simulink model "PassangerVehicle"  (R2022a)
settings: Solver=ode23tb  StartTime=0.0  StopTime=15  RelTol=1e-3
values from neighbouring files (symbols this model uses):
  AccPwrbp = [0 3.0779560993538198]    [Init_Parameters.m]
  AccSpdbp = [256.49641719585139 641.24104298962845]    [Init_Parameters.m]
  InitialLatPosition = 0    [Init_Parameters.m]
  numWheels = 4    [Init_Parameters.m]    (also in VehicleParameters.m)
  TrackWidth = VEH.TrackWidth    [Init_Parameters.m]
  Trans = data.Trans    [Init_Parameters.m]    (also in ModelWorkspace.mat = )
  VEH = data.VEH    [Init_Parameters.m]    (also in ModelWorkspace.mat = ; VehicleParameters.m)
  wheelB = VEH.FrontAxlePositionfromCG+VEH.RearAxlePositionfromCG    [Init_Parameters.m]    (also in VehicleParameters.m)
libraries: autolibutils x6, sharedtransform x5, autolibsharedcoupling x3, vehdynlibsuspension x2, shared6dof x2, autolibsharedtransfixedgear x1, vehdynlibsteering x1, autolibshareddiff x1, autolibsharedmappedengines x1, vehdynlibeom x1, vehdynlibtire x1, vehdynlibtirecommon x1
(part 1 of 4)
settings Model: Creator=monic  LastModifiedBy=monic
settings DebuggingCC: UnconnectedInputMsg=warning  UnconnectedOutputMsg=warning  UnconnectedLineMsg=warning
settings RTWCC: DLArmComputeVersion=19.05

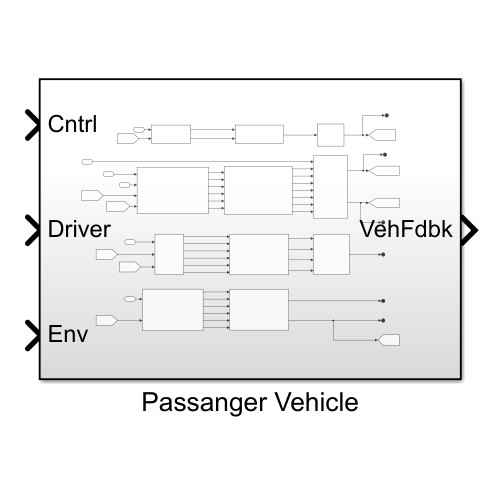
[thumbnail: Simulink's stored preview of the top-level diagram]
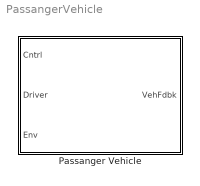
== system PassangerVehicle ==
  Passanger Vehicle : Subsystem

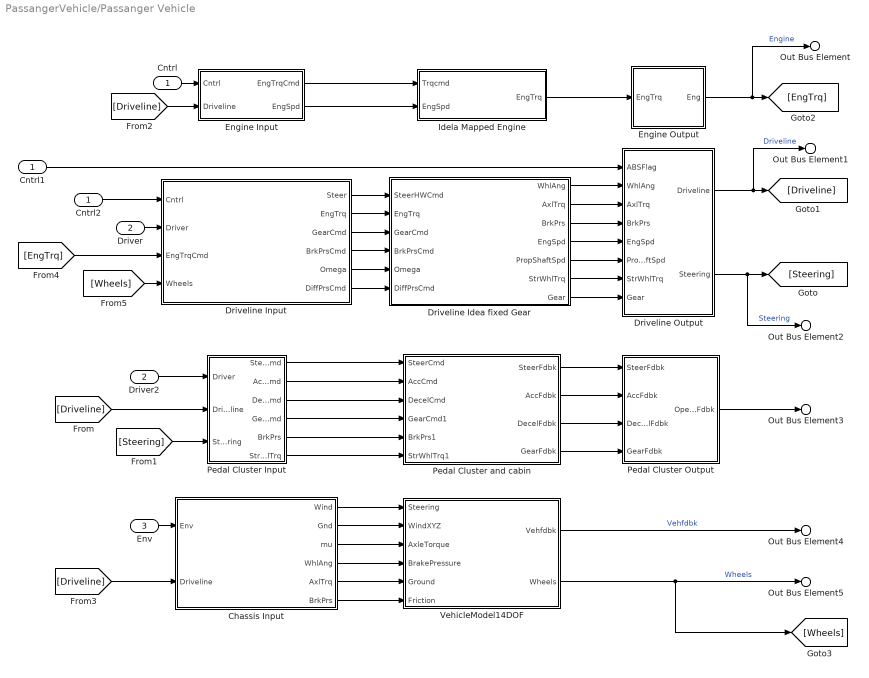
== system PassangerVehicle/Passanger Vehicle ==
  Cntrl : Inport
  Driver : Inport  Port=2
  Env : Inport  Port=3
  Chassis Input : Subsystem
  Cntrl1 : InportShadow
  Cntrl2 : InportShadow
  Driveline Idea fixed Gear : Subsystem
  Driveline Input : Subsystem
  Driveline Output : Subsystem
  Driver2 : InportShadow  Port=2
  Engine Input : Subsystem
  Engine Output : Subsystem
  Idela Mapped Engine : Subsystem
  Pedal Cluster Input : Subsystem
  Pedal Cluster Output : Subsystem
  Pedal Cluster and cabin : Subsystem
  VehicleModel14DOF : Subsystem
  Out Bus Element4 : Outport  PortName=VehFdbk  Element=Body
  Out Bus Element5 : Outport  PortName=VehFdbk  Element=Wheels
  Out Bus Element3 : Outport  PortName=VehFdbk  Element=Driver
  Out Bus Element2 : Outport  PortName=VehFdbk  Element=Steering
  Out Bus Element1 : Outport  PortName=VehFdbk  Element=Driveline
  Out Bus Element : Outport  PortName=VehFdbk  Element=Engine
  wires:
  Driveline Idea fixed Gear/7(Gear) -> Driveline Output/8(Gear)
  [Driveline] -> Chassis Input/2(Driveline)
  Engine Input/1(EngTrqCmd) -> Idela Mapped Engine/1(Trqcmd)
  Pedal Cluster and cabin/2(AccFdbk) -> Pedal Cluster Output/2(AccFdbk)
  Chassis Input/6(BrkPrs) -> VehicleModel14DOF/6(Friction)
  Driveline Input/4(BrkPrsCmd) -> Driveline Idea fixed Gear/4(BrkPrsCmd)
  Pedal Cluster Input/3(DecelCmd) -> Pedal Cluster and cabin/3(DecelCmd)
  VehicleModel14DOF/2(Wheels) -> Out Bus Element5/1, [Wheels]  "Wheels"
  Chassis Input/4(WhlAng) -> VehicleModel14DOF/4(BrakePressure)
  Pedal Cluster Input/2(AccelCmd) -> Pedal Cluster and cabin/2(AccCmd)
  Driver/1 -> Driveline Input/2(Driver)
  Pedal Cluster and cabin/3(DecelFdbk) -> Pedal Cluster Output/3(DecelFdbk)
  Engine Input/2(EngSpd) -> Idela Mapped Engine/2(EngSpd)
  [Driveline] -> Pedal Cluster Input/2(Driveline)
  Driveline Idea fixed Gear/1(WhlAng) -> Driveline Output/2(WhlAng)
  Pedal Cluster and cabin/4(GearFdbk) -> Pedal Cluster Output/4(GearFdbk)
  Driveline Input/3(GearCmd) -> Driveline Idea fixed Gear/3(GearCmd)
  [Steering] -> Pedal Cluster Input/3(Steering)
  Cntrl1/1 -> Driveline Output/1(ABSFlag)
  [EngTrq] -> Driveline Input/3(EngTrqCmd)
  Chassis Input/3(mu) -> VehicleModel14DOF/3(AxleTorque)
  Chassis Input/5(AxlTrq) -> VehicleModel14DOF/5(Ground)
  Driveline Input/6(DiffPrsCmd) -> Driveline Idea fixed Gear/6(DiffPrsCmd)
  Driver2/1 -> Pedal Cluster Input/1(Driver)
  Idela Mapped Engine/1(EngTrq) -> Engine Output/1("EngTrq ")
  Pedal Cluster Input/1(SteerCmd) -> Pedal Cluster and cabin/1(SteerCmd)
  Cntrl/1 -> Engine Input/1(Cntrl)
  Pedal Cluster Input/5(BrkPrs) -> Pedal Cluster and cabin/5(BrkPrs1)
  [Wheels] -> Driveline Input/4(Wheels)
  Driveline Input/1(Steer) -> Driveline Idea fixed Gear/1(SteerHWCmd)
  Driveline Input/2(EngTrq) -> Driveline Idea fixed Gear/2(EngTrq)
  Pedal Cluster and cabin/1(SteerFdbk) -> Pedal Cluster Output/1(SteerFdbk)
  Driveline Input/5(Omega) -> Driveline Idea fixed Gear/5(Omega)
  Env/1 -> Chassis Input/1(Env)
  Driveline Idea fixed Gear/3(BrkPrs) -> Driveline Output/4(BrkPrs)
  Chassis Input/1(Wind) -> VehicleModel14DOF/1(Steering)
  Driveline Idea fixed Gear/4(EngSpd) -> Driveline Output/5(EngSpd)
  Chassis Input/2(Gnd) -> VehicleModel14DOF/2(WindXYZ)
  Driveline Output/2(Steering) -> Out Bus Element2/1, [Steering]  "Steering"
  Engine Output/1(Eng) -> Out Bus Element/1, [EngTrq]  "Engine"
  Driveline Idea fixed Gear/6(StrWhlTrq) -> Driveline Output/7(StrWhlTrq)
  Driveline Idea fixed Gear/5(PropShaftSpd) -> Driveline Output/6(PropShftSpd)
  [Driveline] -> Engine Input/2(Driveline)
  Pedal Cluster Input/4(GearCmd) -> Pedal Cluster and cabin/4(GearCmd1)
  Driveline Idea fixed Gear/2(AxlTrq) -> Driveline Output/3(AxlTrq)
  VehicleModel14DOF/1(Vehfdbk) -> Out Bus Element4/1  "Vehfdbk"
  Pedal Cluster Input/6(StrWhlTrq) -> Pedal Cluster and cabin/6(StrWhlTrq1)
  Cntrl2/1 -> Driveline Input/1(Cntrl)
  Pedal Cluster Output/1(OperatorFdbk) -> Out Bus Element3/1
  Driveline Output/1(Driveline) -> Out Bus Element1/1, [Driveline]  "Driveline"

== system PassangerVehicle/Passanger Vehicle/Chassis Input ==
  Env : Inport
  Driveline : Inport  Port=2
  Bus Selector1 : BusSelector  OutputSignals=Gnd.z.G_FL_z,Gnd.z.G_FR_z,Gnd.z.G_RL_z,Gnd.z.G_RR_z
  Bus Selector2 : BusSelector  OutputSignals=Wind
  Bus Selector3 : BusSelector  OutputSignals=Gnd.mu.mu_FL,Gnd.mu.mu_FR,Gnd.mu.mu_RL,Gnd.mu.mu_RR
  Bus Selector4 : BusSelector  OutputSignals=WhlAng,AxlTrq,BrkPrs
  Vector Concatenate : Concatenate  NumInputs=4
  Vector Concatenate1 : Concatenate  NumInputs=4
  Wind : Outport  VectorParamsAs1DForOutWhenUnconnected=off
  Gnd : Outport  Port=2  VectorParamsAs1DForOutWhenUnconnected=off
  mu : Outport  Port=3  VectorParamsAs1DForOutWhenUnconnected=off
  WhlAng : Outport  Port=4  VectorParamsAs1DForOutWhenUnconnected=off
  AxlTrq : Outport  Port=5  VectorParamsAs1DForOutWhenUnconnected=off
  BrkPrs : Outport  Port=6  VectorParamsAs1DForOutWhenUnconnected=off
  wires:
  Env/1 -> Bus Selector3/1, Bus Selector1/1, Bus Selector2/1
  Bus Selector2/1 -> Wind/1  "<Wind>"
  Bus Selector3/1 -> Vector Concatenate/1  "<mu_FL>"
  Bus Selector3/2 -> Vector Concatenate/2  "<mu_FR>"
  Bus Selector3/3 -> Vector Concatenate/3  "<mu_RL>"
  Bus Selector3/4 -> Vector Concatenate/4  "<mu_RR>"
  Vector Concatenate/1 -> mu/1
  Bus Selector1/1 -> Vector Concatenate1/1  "<G_FL_z>"
  Bus Selector1/2 -> Vector Concatenate1/2  "<G_FR_z>"
  Bus Selector1/3 -> Vector Concatenate1/3  "<G_RL_z>"
  Bus Selector1/4 -> Vector Concatenate1/4  "<G_RR_z>"
  Vector Concatenate1/1 -> Gnd/1
  Driveline/1 -> Bus Selector4/1
  Bus Selector4/2 -> AxlTrq/1  "<AxlTrq>"
  Bus Selector4/1 -> WhlAng/1  "<WhlAng>"
  Bus Selector4/3 -> BrkPrs/1  "<BrkPrs>"

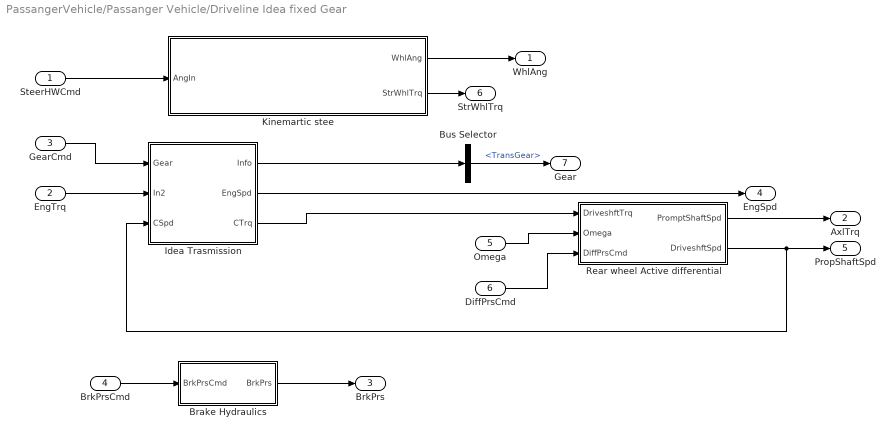
== system PassangerVehicle/Passanger Vehicle/Driveline Idea fixed Gear ==
  SteerHWCmd : Inport
  EngTrq : Inport  Port=2
  GearCmd : Inport  Port=3
  BrkPrsCmd : Inport  Port=4  PortDimensions=4
  Omega : Inport  Port=5
  DiffPrsCmd : Inport  Port=6
  Brake Hydraulics : Subsystem
  Bus Selector : BusSelector  OutputSignals=Trans.TransGear
  Idea Trasmission : Subsystem
  Kinemartic stee : Subsystem
  Rear wheel Active differential : Subsystem
  WhlAng : Outport  Unit=rad  VectorParamsAs1DForOutWhenUnconnected=off
  AxlTrq : Outport  Port=2  VectorParamsAs1DForOutWhenUnconnected=off
  BrkPrs : Outport  Port=3  PortDimensions=4  VectorParamsAs1DForOutWhenUnconnected=off
  EngSpd : Outport  Port=4  VectorParamsAs1DForOutWhenUnconnected=off
  PropShaftSpd : Outport  Port=5  VectorParamsAs1DForOutWhenUnconnected=off
  StrWhlTrq : Outport  Port=6  Unit=N*m  VectorParamsAs1DForOutWhenUnconnected=off
  Gear : Outport  Port=7
  wires:
  Rear wheel Active differential/1(PromptShaftSpd) -> AxlTrq/1
  Omega/1 -> Rear wheel Active differential/2(Omega)
  Rear wheel Active differential/2(DriveshftSpd) -> PropShaftSpd/1, Idea Trasmission/3(CSpd)
  Idea Trasmission/3(CTrq) -> Rear wheel Active differential/1(DriveshftTrq)
  DiffPrsCmd/1 -> Rear wheel Active differential/3(DiffPrsCmd)
  Brake Hydraulics/1(BrkPrs) -> BrkPrs/1
  Idea Trasmission/2(EngSpd) -> EngSpd/1
  BrkPrsCmd/1 -> Brake Hydraulics/1(BrkPrsCmd)
  GearCmd/1 -> Idea Trasmission/1(Gear)
  SteerHWCmd/1 -> Kinemartic stee/1(AngIn)
  Idea Trasmission/1(Info) -> Bus Selector/1
  Kinemartic stee/2(StrWhlTrq) -> StrWhlTrq/1
  Kinemartic stee/1(WhlAng) -> WhlAng/1
  EngTrq/1 -> Idea Trasmission/2(In2)
  Bus Selector/1 -> Gear/1  "<TransGear>"

== system PassangerVehicle/Passanger Vehicle/Driveline Input ==
  Cntrl : Inport
  Driver : Inport  Port=2
  EngTrqCmd : Inport  Port=3
  Wheels : Inport  Port=4
  Bus Selector1 : BusSelector  OutputSignals=SteerCmd
  Bus Selector2 : BusSelector  OutputSignals=TireFrame.Omega
  Bus Selector3 : BusSelector  OutputSignals=Transmission.GearCmd,Brake.BrkPrsCmd,Diff.DiffPrsCmd
  Bus Selector4 : BusSelector  OutputSignals=EngTrq
  Data Type Conversion : DataTypeConversion  SaturateOnIntegerOverflow=off  RndMeth=Floor
  Steer : Outport  VectorParamsAs1DForOutWhenUnconnected=off
  EngTrq : Outport  Port=2  VectorParamsAs1DForOutWhenUnconnected=off
  GearCmd : Outport  Port=3  VectorParamsAs1DForOutWhenUnconnected=off
  BrkPrsCmd : Outport  Port=4  VectorParamsAs1DForOutWhenUnconnected=off
  Omega : Outport  Port=5  VectorParamsAs1DForOutWhenUnconnected=off
  DiffPrsCmd : Outport  Port=6  VectorParamsAs1DForOutWhenUnconnected=off
  wires:
  Cntrl/1 -> Bus Selector3/1
  Bus Selector3/1 -> Data Type Conversion/1  "<GearCmd>"
  Driver/1 -> Bus Selector1/1
  Wheels/1 -> Bus Selector2/1
  Bus Selector2/1 -> Omega/1  "<Omega>"
  Bus Selector3/2 -> BrkPrsCmd/1  "<BrkPrsCmd>"
  EngTrqCmd/1 -> Bus Selector4/1
  Bus Selector1/1 -> Steer/1  "<SteerCmd>"
  Bus Selector4/1 -> EngTrq/1  "<EngTrq>"
  Bus Selector3/3 -> DiffPrsCmd/1  "<DiffPrsCmd>"
  Data Type Conversion/1 -> GearCmd/1

== system PassangerVehicle/Passanger Vehicle/Driveline Output ==
  ABSFlag : Inport
  WhlAng : Inport  Port=2
  AxlTrq : Inport  Port=3
  BrkPrs : Inport  Port=4
  EngSpd : Inport  Port=5
  PropShftSpd : Inport  Port=6
  StrWhlTrq : Inport  Port=7
  Gear : Inport  Port=8
  Bus Creator1 : BusCreator  Inputs=7
  Bus Creator2 : BusCreator  Inputs=1
  Driveline : Outport  VectorParamsAs1DForOutWhenUnconnected=off
  Steering : Outport  Port=2  VectorParamsAs1DForOutWhenUnconnected=off
  wires:
  Bus Creator1/1 -> Driveline/1  "Driveline"
  PropShftSpd/1 -> Bus Creator1/5  "PropShftSpd"
  AxlTrq/1 -> Bus Creator1/2  "AxlTrq"
  WhlAng/1 -> Bus Creator1/1  "WhlAng"
  EngSpd/1 -> Bus Creator1/4  "EngSpd"
  BrkPrs/1 -> Bus Creator1/3  "BrkPrs"
  StrWhlTrq/1 -> Bus Creator2/1  "StrWhlTrq"
  Bus Creator2/1 -> Steering/1  "Steering"
  Gear/1 -> Bus Creator1/6  "Gear"
  ABSFlag/1 -> Bus Creator1/7  "ABSFlag"

== system PassangerVehicle/Passanger Vehicle/Engine Input ==
  Cntrl : Inport
  Driveline : Inport  Port=2
  Bus Selector : BusSelector  OutputSignals=ECU.EngTrqCmd
  Bus Selector1 : BusSelector  OutputSignals=EngSpd
  EngTrqCmd : Outport  VectorParamsAs1DForOutWhenUnconnected=off
  EngSpd : Outport  Port=2  VectorParamsAs1DForOutWhenUnconnected=off
  wires:
  Driveline/1 -> Bus Selector1/1
  Cntrl/1 -> Bus Selector/1
  Bus Selector/1 -> EngTrqCmd/1  "<EngTrqCmd>"
  Bus Selector1/1 -> EngSpd/1  "<EngSpd>"

== system PassangerVehicle/Passanger Vehicle/Engine Output ==
  "EngTrq " : Inport
  Bus Creator : BusCreator  Inputs=1
  Eng : Outport  VectorParamsAs1DForOutWhenUnconnected=off
  wires:
  "EngTrq "/1 -> Bus Creator/1  "EngTrq"
  Bus Creator/1 -> Eng/1
